simulink model "OpenLoop_2021a"  (R2022a)
settings: Solver=ode15s  StartTime=0.0  StopTime=500000  RelTol=1e-6  AbsTol=1e-8
undefined symbols (not defined in the file or in its folder): in, sigbuilder_block
settings Model: SimulationMode=accelerator  Creator=Sergio  LastModifiedBy=LADES
settings SolverCC: AutoScaleAbsTol=off
settings DataIOCC: SaveFormat=Array  ReturnWorkspaceOutputs=off
settings DebuggingCC: AlgebraicLoopMsg=none  UnconnectedInputMsg=warning  UnconnectedOutputMsg=warning  UnconnectedLineMsg=warning
settings RTWCC: DLArmComputeVersion=19.05

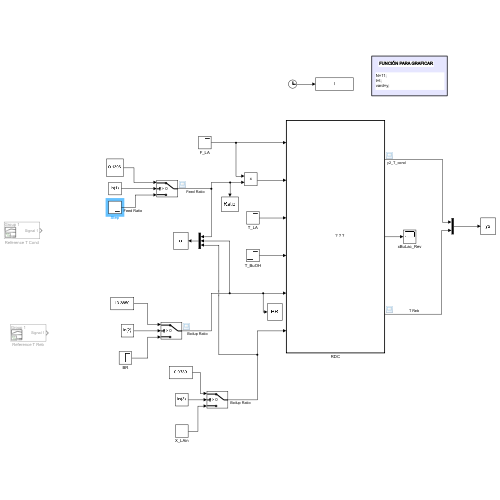
[thumbnail: Simulink's stored preview of the top-level diagram]
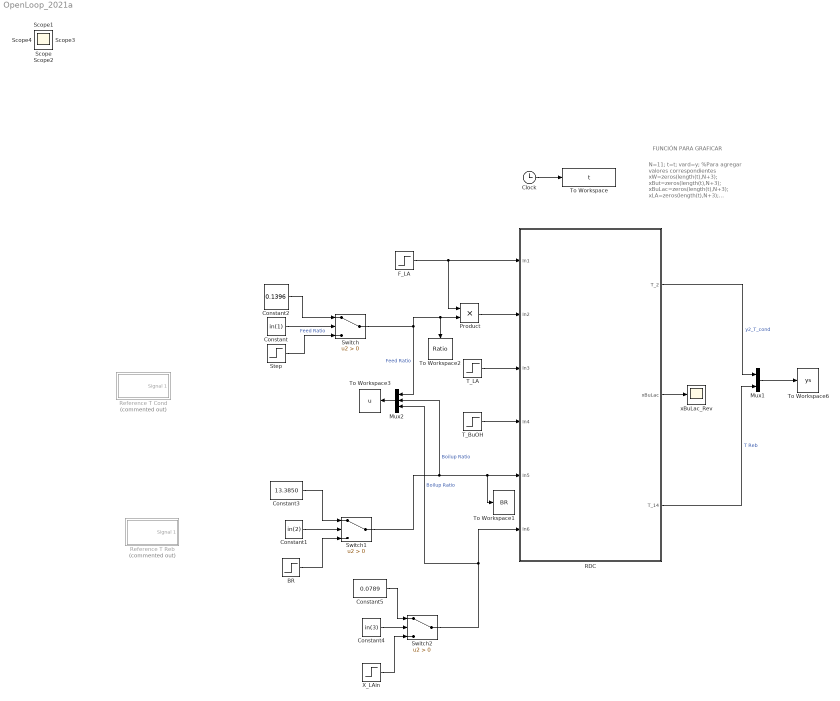
== system OpenLoop_2021a ==
  note: FUNCIÓN PARA GRAFICAR
  note: N=11;
      | t=t;
      | vard=y;
      |
      | %Para agregar valores correspondientes
      | xW=zeros(length(t),N+3); xBut=zeros(length(t),N+3); xBuLac=zeros(length(t),N+3); xLA=zeros(length(t),N+3); Z=zeros(length(t),N+3); ZW=zeros(length(t),N+3);ZBut=zeros(length(t),N+3);ZBuLac=zeros(length(t),N+3);ZLA=zeros(length(t),N+3);T=zeros(length(t),N+3);
      | for i=1:1:N+3
      | Z(:,i)=vard(:,i);
      | ZW(:,i)=vard(:,(N+3)+i);
      | ZBut(:,i)=vard(:,2*(N+3)+i);
      | ZBuLac(:,i)=vard(:,3*(N+3)+i);
      | ZLA(:,i)=vard(:,4*(N+3)+i);
      | T(:,i)=vard(:,5*(N+3)+i);
      | end
      | Z=transpose(Z);
      | ZW=transpose(ZW);
      | ZBut=transpose(ZBut);
      | ZBuLac=transpose(ZBuLac);
      | ZLA=transpose(ZLA);
      | T=transpose(T);
      | %Fracciones molares
      | xW=ZW./Z;
      | xBut=ZBut./Z;
      | xBuLac=ZBuLac./Z;
      | xLA=ZLA./Z;
      |
      | flat=1:N+3;
      | flat=flat';
      | figure(1);subplot(2,1,1);plot(flat,xW(:,end), flat,xBut(:,end), flat, xBuLac(:,end),flat, xLA(:,end));xlabel( 'Stages' );ylabel( 'Molar Frac %' );
      | legend( 'xW' , 'xBut' , 'xBuLac' , 'xLA' ); axis([1 N+3 0 1]);
      | subplot(2,1,2);plot(flat,T(:,end));xlabel( 'Stages' );ylabel( 'Temperature (K)' ); axis([1 N+3 min(T(:,end)) max(T(:,end))]);
  BR : Step  Time=25*3600  Before=13.3850  After=26.77  SampleTime=0
  Clock : Clock
  Constant : Constant  Value=in(1)
  Constant1 : Constant  Value=in(2)
  Constant2 : Constant  Value=0.1396
  Constant3 : Constant  Value=13.3850
  Constant4 : Constant  Value=in(3)
  Constant5 : Constant  Value=0.0789
  F_LA : Step  Time=0  Before=4.7366E-05  After=4.7366E-05  SampleTime=0
  Mux1 : Mux  Inputs=2
  Mux2 : Mux  Inputs=3
  Product : Product
  RDC : Subsystem  TreatAsAtomicUnit=on
      mask Display: image('RDC_1.jpg'); % Use "Edit Image" on toolstrip to change.
  Reference T Cond : Subsystem  Tag=STV Subsys  Commented=on  LoadFcn=sigbuilder_block('load');  StartFcn=sigbuilder_block('start');  StopFcn=sigbuilder_block('stop');  ClipboardFcn=sigbuilder_block('clipboard');  mask(Sigbuilder block){tuvar=[0:10]}
      mask help: Simulink:masks:SigbuilderBlock_MD
      mask init:
      | if ~strcmp(get_param(bdroot(gcbh),'SimulationStatus'),'stopped') tuvar = sigbuilder_block('maskInit'); end
      settings: CopyFcn=sigbuilder_block('copy');  DeleteFcn=sigbuilder_block('delete');  ModelCloseFcn=sigbuilder_block('modelClose');  PreSaveFcn=sigbuilder_block('preSave');  PauseFcn=sigbuilder_block('pause');  ContinueFcn=sigbuilder_block('continue');  NameChangeFcn=sigbuilder_block('namechange');  OpenFcn=sigbuilder_block('open',[0 30 1024.5 488.25 ]);  CloseFcn=sigbuilder_block('close');
      mask Display: plot(0, 0, 100, 100,[2, 2, 32, 32, 2], [68, 8, 8, 68, 68],[32, 2], [38, 38], [32, 19, 2],[53, 60, 44], [32, 17, 17, 2],[16, 16, 31, 31]);txt = getActiveGroup(gcbh);text(2, 100, txt,'verticalAlignment', 'top');
  Reference T Reb : Subsystem  Tag=STV Subsys  Commented=on  LoadFcn=sigbuilder_block('load');  StartFcn=sigbuilder_block('start');  StopFcn=sigbuilder_block('stop');  ClipboardFcn=sigbuilder_block('clipboard');  mask(Sigbuilder block){tuvar=[0:10]}
      mask help: Simulink:masks:SigbuilderBlock_MD
      mask init:
      | if ~strcmp(get_param(bdroot(gcbh),'SimulationStatus'),'stopped') tuvar = sigbuilder_block('maskInit'); end
      settings: CopyFcn=sigbuilder_block('copy');  DeleteFcn=sigbuilder_block('delete');  ModelCloseFcn=sigbuilder_block('modelClose');  PreSaveFcn=sigbuilder_block('preSave');  PauseFcn=sigbuilder_block('pause');  ContinueFcn=sigbuilder_block('continue');  NameChangeFcn=sigbuilder_block('namechange');  OpenFcn=sigbuilder_block('open',[-1363.8 -35.4 1141.2 501 ]);  CloseFcn=sigbuilder_block('close');
      mask Display: plot(0, 0, 100, 100,[2, 2, 32, 32, 2], [68, 8, 8, 68, 68],[32, 2], [38, 38], [32, 19, 2],[53, 60, 44], [32, 17, 17, 2],[16, 16, 31, 31]);txt = getActiveGroup(gcbh);text(2, 100, txt,'verticalAlignment', 'top');
  Step : Step  Time=25*3600  Before=0.1396  After=0.1317  SampleTime=0
  Switch : Switch  Criteria=u2 > Threshold  SaturateOnIntegerOverflow=off  InputSameDT=off
  Switch1 : Switch  Criteria=u2 > Threshold  SaturateOnIntegerOverflow=off  InputSameDT=off
  Switch2 : Switch  Criteria=u2 > Threshold  SaturateOnIntegerOverflow=off  InputSameDT=off
  T_BuOH : Step  Time=0  Before=90  After=90  SampleTime=0
  T_LA : Step  Time=0  Before=80  After=80  SampleTime=0
  To Workspace : ToWorkspace  VariableName=t  SampleTime=100
  To Workspace1 : ToWorkspace  VariableName=BR
  To Workspace2 : ToWorkspace  VariableName=Ratio
  To Workspace3 : ToWorkspace  VariableName=u  SampleTime=100
  To Workspace6 : ToWorkspace  VariableName=ys  SampleTime=100
  X_LAin : Step  Time=25*3600  Before=0.0789  After=0.0789*1.1  SampleTime=0
  xBuLac_Rev : Scope
  Scope{,1..4} (5 alike) : Scope
  wires:
  Mux1/1 -> To Workspace6/1
  Clock/1 -> To Workspace/1
  Switch1/1 -> Mux2/2, RDC/5(In5), To Workspace1/1  "Boilup Ratio"
  RDC/3(T_14) -> Mux1/2  "T Reb"
  RDC/1(T_2) -> Mux1/1  "y2_T_cond"
  RDC/2(xBuLac) -> xBuLac_Rev/1
  T_LA/1 -> RDC/3(In3)
  T_BuOH/1 -> RDC/4(In4)
  F_LA/1 -> Product/1, RDC/1(In1)
  Product/1 -> RDC/2(In2)
  Switch/1 -> Mux2/1, To Workspace2/1, Product/2  "Feed Ratio"
  Constant/1 -> Switch/2
  Constant1/1 -> Switch1/2
  X_LAin/1 -> Switch2/3
  Mux2/1 -> To Workspace3/1
  Constant2/1 -> Switch/1
  Step/1 -> Switch/3  "Feed Ratio"
  BR/1 -> Switch1/3
  Constant3/1 -> Switch1/1
  Switch2/1 -> Mux2/3, RDC/6(In6)  "Boilup Ratio"
  Constant4/1 -> Switch2/2
  Constant5/1 -> Switch2/1

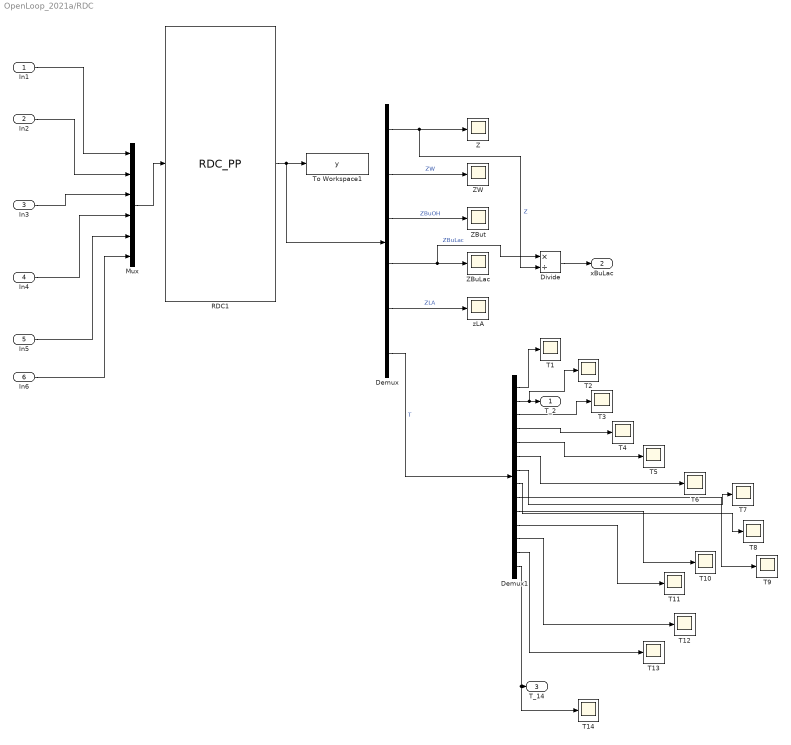
== system OpenLoop_2021a/RDC ==
  In1 : Inport
  In2 : Inport  Port=2
  In3 : Inport  Port=3
  In4 : Inport  Port=4
  In5 : Inport  Port=5
  In6 : Inport  Port=6
  Demux : Demux  Outputs=6
  Demux1 : Demux  Outputs=14
  Divide : Product  Inputs=*/
  Mux : Mux  Inputs=6
  RDC1 : M-S-Function  FunctionName=RDC_PP  Parameters=0.0294255399999924, 0.0811704339705782, 0.0162707977782127, 0.0152195188871099, 0.0224867496465455, 0.0182567192037436, 0.0128131806843584, 0.0105610404844501, 0.0100295910766296, 0.00989902199616042, 0.00985506895369427, 0.00972353786294072, 0.00929737378000563, 0.0740075214052103, 0.0206796389999989, 0.0630951565828122, 0.00928016546563196, 0.00809300923899119, 0.0163652354182154, 0.0108347821650824, 0.00383299640629196, 0.000935315019408970, 0.000215555762486145, 4.87789841749069e-05, 1.11021457187585e-05, 2.61803316035419e-06, 7.20186608045705e-07, 1.35374534697822e-06, 0.00874584599999762, 0.0180752722830340, 0.00699053197065110, 0.00711845663343252, 0.00522785656979894, 0.00666765005243259, 0.00839807821941969, 0.00913419726834427, 0.00933939401622277, 0.00937473053558701, 0.00934494106239325, 0.00903735150603872, 0.00723351567277999, 0.0248033653146468, 5.23999999999949e-08, 4.81484156950321e-09, 7.14107501602844e-08, 2.31516316317851e-06, 7.62365054263931e-05, 0.000128175084101672, 0.000234530145778035, 0.000383575237042647, 0.000365751828354146, 0.000363692233830313, 0.000377204158907935, 0.000515587507629627, 0.00161145368645164, 0.0396929517641084, 2.55000000000013e-09, 2.89890380623561e-10, 2.89311795036437e-08, 5.73785152304380e-06, 0.000817421153104752, 0.000626111902126832, 0.000347575912868740, 0.000107952959654228, 0.000108889469566514, 0.000111820242568191, 0.000121821586674327, 0.000167980816112021, 0.000451684234165955, 0.00950985058110795, 325.752539411885, 359.855171896379, 359.855171896394, 360.365953255051, 378.707862062715, 379.183184764873, 379.616042109027, 379.518439647629, 382.113127317567, 382.743812903949, 383.445761034128, 384.918883937602, 392.520953801984, 407.258683188477
      mask Display: image('RDC.JPG'); % Use "Edit Image" on toolstrip to change.
  T{1..14} (14 alike) : Scope
  To Workspace1 : ToWorkspace  VariableName=y
  Z : Scope
  ZBuLac : Scope
  ZBut : Scope
  ZW : Scope
  zLA : Scope
  T_2 : Outport
  xBuLac : Outport  Port=2
  T_14 : Outport  Port=3
  wires:
  Demux/5 -> zLA/1  "ZLA"
  In2/1 -> Mux/2
  RDC1/1 -> Demux/1, To Workspace1/1
  In1/1 -> Mux/1
  Mux/1 -> RDC1/1
  Demux/1 -> Divide/2, Z/1  "Z"
  In4/1 -> Mux/4
  In3/1 -> Mux/3
  In5/1 -> Mux/5
  Demux/2 -> ZW/1  "ZW"
  Demux/6 -> Demux1/1  "T"
  Demux/4 -> Divide/1, ZBuLac/1  "ZBuLac"
  Demux/3 -> ZBut/1  "ZBuOH"
  Demux1/2 -> T2/1, T_2/1
  Demux1/14 -> T14/1, T_14/1
  Demux1/1 -> T1/1
  Demux1/3 -> T3/1
  Demux1/4 -> T4/1
  Demux1/5 -> T5/1
  Demux1/6 -> T6/1
  Demux1/7 -> T7/1
  Demux1/8 -> T8/1
  Demux1/9 -> T9/1
  Demux1/10 -> T10/1
  Demux1/11 -> T11/1
  Demux1/12 -> T12/1
  Demux1/13 -> T13/1
  Divide/1 -> xBuLac/1
  In6/1 -> Mux/6

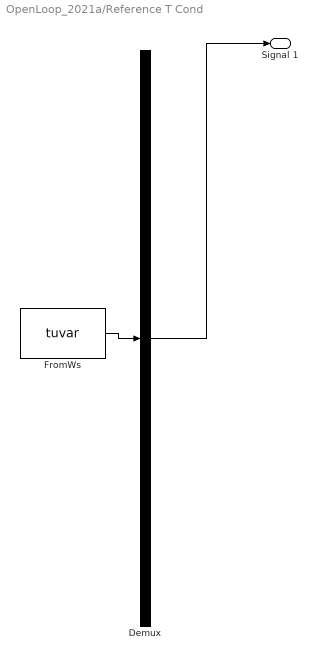
== system OpenLoop_2021a/Reference T Cond ==
  Demux : Demux  Tag=STV Demux  Outputs=1
      settings: DisplayOption=none
  FromWs : FromWorkspace  Tag=STV FromWs  VariableName=tuvar
      SigBuilderData=|
      | common.afterFinalStr = 'Extrapolate'
      | common.sampleTime = 0
      | dataSet(1).timeRange = [0 720000]
      | dataSet(1).name = 'Group 1'
      | dataSet(2).timeRange = [0 720000]
      | dataSet(2).name = 'Group 2'
      | sbobj.Groups(1).Name = 'Group 1'
      | sbobj.Groups(1).Signals.Name = 'Signal 1'
      | sbobj.Groups(1).Signals.XData = [0 10000 10000 25000 25000 35000 35000 40000 40000 45000 45000 50000 50001 720000]
      | sbobj.Groups(1).Signals.YData = [0.1317 0.1317 0.139 0.139 0.1317 0.1317 0.139 0.139 0.1317 0.1317 0.139 0.139 0.1317 0.1317]
      | sbobj.Groups(1).TimeRange = [0 720000]
      | sbobj.Groups(2).Name = 'Group 2'
      | sbobj.Groups(2).Signals.Name = 'Signal 1'
      | sbobj.Groups(2).Signals.XData = [0 10000 10000 25000 25000 35000 35000 40000 40000 45000 45000 50000 50001 720000]
      | sbobj.Groups(2).Signals.YData = [0.1317 0.1317 0.139 0.139 0.1317 0.1317 0.139 0.139 0.1317 0.1317 0.139 0.139 0.1317 0.1317]
      | sbobj.Groups(2).TimeRange = [0 720000]
  Signal 1 : Outport  Tag=STV Outport
  wires:
  FromWs/1 -> Demux/1
  Demux/1 -> Signal 1/1

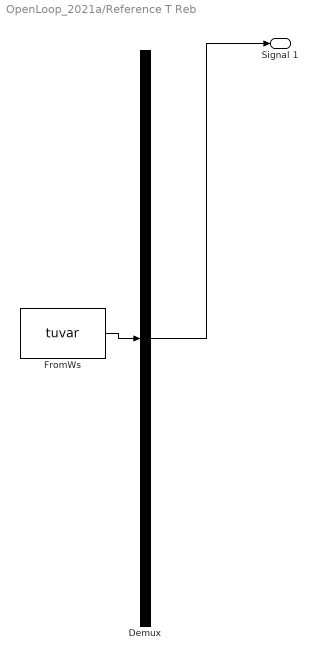
== system OpenLoop_2021a/Reference T Reb ==
  Demux : Demux  Tag=STV Demux  Outputs=1
      settings: DisplayOption=none
  FromWs : FromWorkspace  Tag=STV FromWs  VariableName=tuvar
      SigBuilderData=|
      | common.afterFinalStr = 'Extrapolate'
      | common.sampleTime = 0
      | dataSet.timeRange = [0 54000]
      | dataSet.name = 'Group 1'
      | sbobj.Groups.Name = 'Group 1'
      | sbobj.Groups.Signals.Name = 'Signal 1'
      | sbobj.Groups.Signals.XData = [0 10000 10000 25000 25000 35000 35000 40000 40000 45000 45000 50000 50001 54000]
      | sbobj.Groups.Signals.YData = [26.77 26.77 25 25 26.77 26.77 25 25 26.77 26.77 25 25 26.77 26.77]
      | sbobj.Groups.TimeRange = [0 54000]
  Signal 1 : Outport  Tag=STV Outport
  wires:
  Demux/1 -> Signal 1/1
  FromWs/1 -> Demux/1
